simulink model "instalatie_cu_filtru_si_perturbatie"  (R2022b)
settings: Solver=VariableStepAuto  StartTime=0.0  StopTime=10.0  RelTol=1e-3
settings Model: Creator=fabian  LastModifiedBy=fabian
settings DebuggingCC: ModelReferenceExtraNoncontSigs=warning

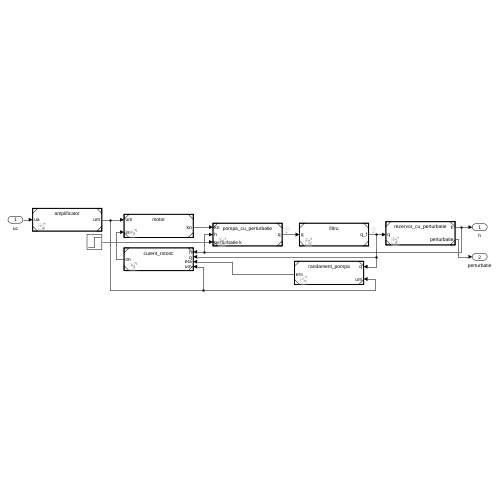
[thumbnail: Simulink's stored preview of the top-level diagram]
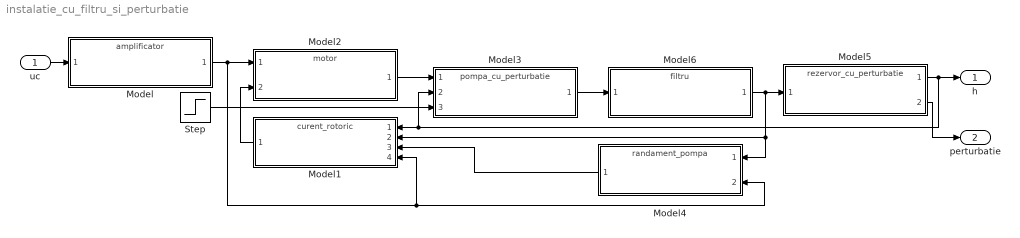
== system instalatie_cu_filtru_si_perturbatie ==
  uc : Inport
  Model : ModelReference  ModelNameDialog=amplificator.slx  SimulationMode=Normal  ModelReferenceVersion=1.1
  Model1 : ModelReference  ModelNameDialog=curent_rotoric.slx  SimulationMode=Normal  ModelReferenceVersion=1.2
  Model2 : ModelReference  ModelNameDialog=motor.slx  SimulationMode=Normal  ModelReferenceVersion=1.1
  Model3 : ModelReference  ModelNameDialog=pompa_cu_perturbatie.slx  SimulationMode=Normal  ModelReferenceVersion=1.1
  Model4 : ModelReference  ModelNameDialog=randament_pompa.slx  SimulationMode=Normal  ModelReferenceVersion=1.2
  Model5 : ModelReference  ModelNameDialog=rezervor_cu_perturbatie.slx  SimulationMode=Normal  ModelReferenceVersion=1.6
  Model6 : ModelReference  ModelNameDialog=filtru.slx  SimulationMode=Normal  ModelReferenceVersion=1.9
  Step : Step  Time=1000  After=0.01  SampleTime=0
  h : Outport
  perturbatie : Outport  Port=2
  wires:
  Model3/1 -> Model6/1
  Model6/1 -> Model4/1, Model1/2, Model5/1
  Model2/1 -> Model3/1
  uc/1 -> Model/1
  Model4/1 -> Model1/3
  Model/1 -> Model2/1, Model1/4, Model4/2
  Model5/1 -> Model3/2, Model1/1, h/1
  Model1/1 -> Model2/2
  Step/1 -> Model3/3
  Model5/2 -> perturbatie/1
